simulink model "she_pwm_c_Bridge"  (R2023b)
settings: Solver=ode23t  StartTime=0.0  StopTime=0.1  MaxStep=1e-6  RelTol=1e-3
model workspace (MAT data in the model file):
  Mf = 48
  Vdc = 48
  ang_converted = 0
  compare_levels = [0 0]
  f = 50
  fs = 48
values from neighbouring files (symbols this model uses):
  angle_levels = zeros(1,angles_no)    [she_pwm.m]
libraries: spsIGBTDiodeLib x20, spsDCVoltageSourceLib x5, simulink x2, spsCurrentMeasurementLib x1, spsSeriesRLCBranchLib x1, spsTHDLib x1, spsVoltageMeasurementLib x1, sps_lib x1
settings Model: Creator=ixale  LastModifiedBy=ixale
settings DataIOCC: ReturnWorkspaceOutputs=off

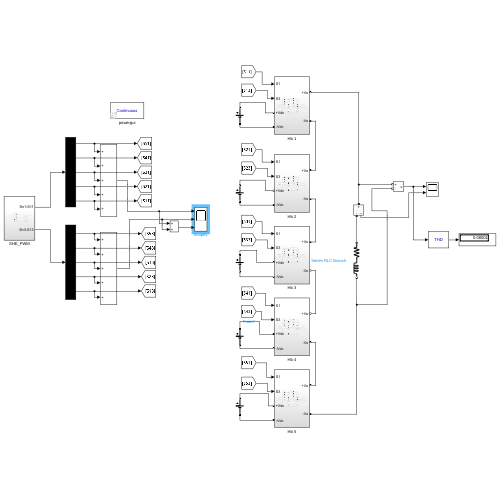
[thumbnail: Simulink's stored preview of the top-level diagram]
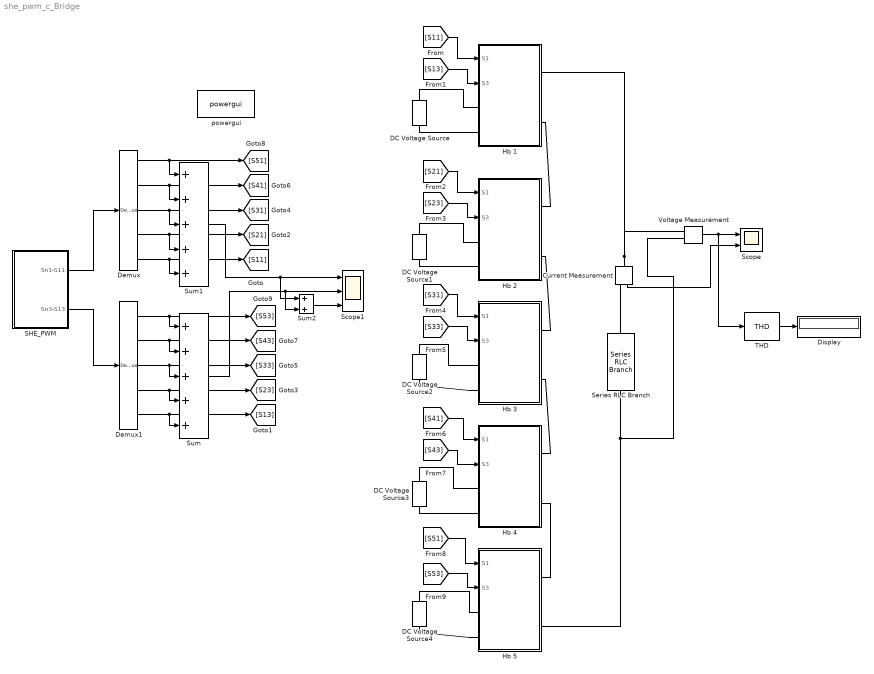
== system she_pwm_c_Bridge ==
  Current Measurement : spsCurrentMeasurementLib/Current Measurement  PhasorSimulation=off  OutputType=Complex  PSBequivalent=0
  DC Voltage Source{,1..4} (5 alike) : spsDCVoltageSourceLib/DC Voltage Source  Amplitude=Vdc  Measurements=None
  Demux : Demux  Outputs=5
  Demux1 : Demux  Outputs=5
  Display : Display
  Hb 1 : Subsystem
  Hb 2 : Subsystem
  Hb 3 : Subsystem
  Hb 4 : Subsystem
  Hb 5 : Subsystem
  SHE_PWM : Subsystem
  Scope : Scope  NumInputPorts=2
  Scope1 : Scope  NumInputPorts=3
  Series RLC Branch : spsSeriesRLCBranchLib/Series RLC Branch  LConnTagsString=__new0  RConnTagsString=__new0  BranchType=RL  Resistance=1  Inductance=1e-3  SetiL0=off  InitialCurrent=0  Capacitance=1e-6  Setx0=off  InitialVoltage=0  Measurements=None
  Sum : Sum  Inputs=+++++
  Sum1 : Sum  Inputs=+++++
  Sum2 : Sum
  THD : spsTHDLib/THD  Freq=50  Ts=0
  Voltage Measurement : spsVoltageMeasurementLib/Voltage Measurement  PhasorSimulation=off  OutputType=Complex  PSBequivalent=0
  powergui : sps_lib/powergui  Priority=1  SimulationMode=Continuous  SampleTime=1e-6  frequency=60  Iterations=50  frequencyindice=0  Pbase=100e6  ErrMax=1e-4  UnitsV=kV  UnitsW=MW  buscounter=0  FunctionMessages=off  echomessages=off  EnableUseOfTLC=off  CurrentSourceSwitches=off  DisableSnubberDevices=off  DisableRonSwitches=off  DisableVfSwitches=off  DisplayEquations=off  AutomaticDiscreteSolvers=off  SolverType=Tustin/Backward Euler (TBE)  Interpol=off  ExternalGateDelay=off  methode=off  Ts=100  x0status=blocks  SPID=on  SwTol=0  HookPort=off  NonlinearTolerance=1e-4  nMaxIteration=100  ContinueOnMaxIteration=off  RestoreLinks=warning  ResistiveCurrentMeasurement=off  Frange=[0:2:500]  Ylog=off  Xlog=on  ShowGrid=off  save=off  variable=ZData  structure=0  ZoomFFT=off  StartTime=0.0  cycles=1  DisplayStyle=1  fundamental=60  FreqAxis=off  MaxFrequency=1000  frequencyindicesteady=1  RmsSteady=1  display=off
  wires:
  Voltage Measurement/1 -> THD/1, Scope/1
  Current Measurement/1 -> Scope/2
  THD/1 -> Display/1
  [S11] -> Hb 1/1(S1)
  [S13] -> Hb 1/2(S3)
  [S23] -> Hb 2/2(S3)
  [S21] -> Hb 2/1(S1)
  [S31] -> Hb 3/1(S1)
  [S33] -> Hb 3/2(S3)
  [S43] -> Hb 4/2(S3)
  [S41] -> Hb 4/1(S1)
  [S51] -> Hb 5/1(S1)
  [S53] -> Hb 5/2(S3)
  SHE_PWM/1(Sn1-S11) -> Demux/1
  SHE_PWM/2(Sn3-S13) -> Demux1/1
  Demux1/3 -> Sum/3, [S33]
  Demux/1 -> Sum1/1, [S51]
  Demux/2 -> Sum1/2, [S41]
  Demux/3 -> Sum1/3, [S31]
  Demux/4 -> Sum1/4, [S21]
  Demux/5 -> Sum1/5, [S11]
  Sum1/1 -> Scope1/1, Sum2/1
  Sum/1 -> Sum2/2, Scope1/2
  Sum2/1 -> Scope1/3
  Demux1/4 -> Sum/4, [S23]
  Demux1/5 -> Sum/5, [S13]
  Demux1/2 -> Sum/2, [S43]
  Demux1/1 -> Sum/1, [S53]
  connections:
  Voltage Measurement/LConn2 -- Hb 5/RConn2 -- Series RLC Branch/RConn1
  Current Measurement/LConn1 -- Hb 1/RConn1 -- Voltage Measurement/LConn1
  Current Measurement/RConn1 -- Series RLC Branch/LConn1
  Hb 1/LConn1 -- DC Voltage Source/RConn1
  Hb 1/LConn2 -- DC Voltage Source/LConn1
  Hb 2/LConn1 -- DC Voltage Source1/RConn1
  Hb 2/LConn2 -- DC Voltage Source1/LConn1
  Hb 3/LConn1 -- DC Voltage Source2/RConn1
  Hb 3/LConn2 -- DC Voltage Source2/LConn1
  Hb 4/LConn1 -- DC Voltage Source3/RConn1
  Hb 4/LConn2 -- DC Voltage Source3/LConn1
  Hb 5/LConn1 -- DC Voltage Source4/RConn1
  Hb 5/LConn2 -- DC Voltage Source4/LConn1
  Hb 2/RConn1 -- Hb 1/RConn2
  Hb 3/RConn1 -- Hb 2/RConn2
  Hb 5/RConn1 -- Hb 4/RConn2
  Hb 4/RConn1 -- Hb 3/RConn2

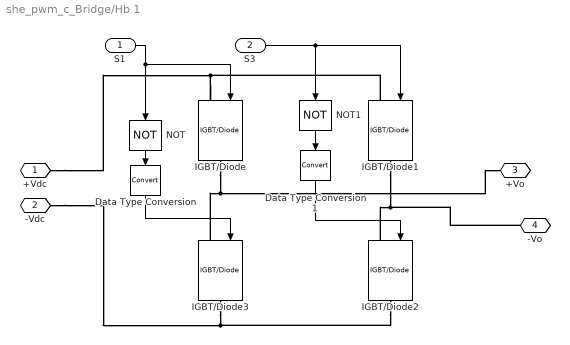
== system she_pwm_c_Bridge/Hb 1 ==
  S1 : Inport
  S3 : Inport  Port=2
  Data Type Conversion : DataTypeConversion  SaturateOnIntegerOverflow=off  RndMeth=Floor
  Data Type Conversion1 : DataTypeConversion  SaturateOnIntegerOverflow=off  RndMeth=Floor
  IGBT/Diode{,1..3} (4 alike) : spsIGBTDiodeLib/IGBT//Diode  Ron=1e-3  Rs=1e5  Cs=inf  Measurements=off
  NOT : Logic  Operator=NOT  IconShape=distinctive  AllPortsSameDT=off  OutDataTypeStr=boolean
  NOT1 : Logic  Operator=NOT  IconShape=distinctive  AllPortsSameDT=off  OutDataTypeStr=boolean
  +Vdc : PMIOPort  Side=Left
  -Vdc : PMIOPort  Port=2  Side=Left
  +Vo : PMIOPort  Port=3  Side=Right
  -Vo : PMIOPort  Port=4  Side=Right
  wires:
  S1/1 -> IGBT/Diode/1, NOT/1
  NOT/1 -> Data Type Conversion/1
  Data Type Conversion/1 -> IGBT/Diode3/1
  Data Type Conversion1/1 -> IGBT/Diode2/1
  NOT1/1 -> Data Type Conversion1/1
  S3/1 -> IGBT/Diode1/1, NOT1/1
  connections:
  IGBT/Diode3/RConn1 -- IGBT/Diode2/RConn1 -- -Vdc/RConn1
  IGBT/Diode1/LConn1 -- +Vdc/RConn1 -- IGBT/Diode/LConn1
  IGBT/Diode3/LConn1 -- IGBT/Diode/RConn1 -- +Vo/RConn1
  IGBT/Diode2/LConn1 -- IGBT/Diode1/RConn1 -- -Vo/RConn1

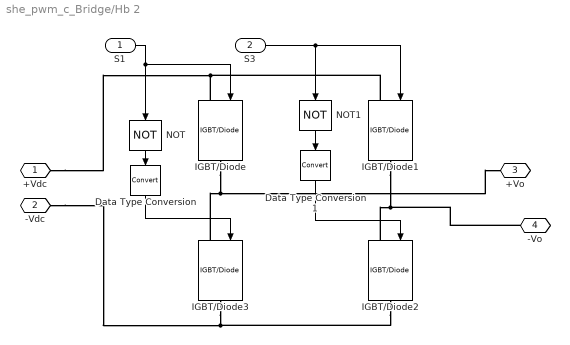
== system she_pwm_c_Bridge/Hb 2 ==
  S1 : Inport
  S3 : Inport  Port=2
  Data Type Conversion : DataTypeConversion  SaturateOnIntegerOverflow=off  RndMeth=Floor
  Data Type Conversion1 : DataTypeConversion  SaturateOnIntegerOverflow=off  RndMeth=Floor
  IGBT/Diode{,1..3} (4 alike) : spsIGBTDiodeLib/IGBT//Diode  Ron=1e-3  Rs=1e5  Cs=inf  Measurements=off
  NOT : Logic  Operator=NOT  IconShape=distinctive  AllPortsSameDT=off  OutDataTypeStr=boolean
  NOT1 : Logic  Operator=NOT  IconShape=distinctive  AllPortsSameDT=off  OutDataTypeStr=boolean
  +Vdc : PMIOPort  Side=Left
  -Vdc : PMIOPort  Port=2  Side=Left
  +Vo : PMIOPort  Port=3  Side=Right
  -Vo : PMIOPort  Port=4  Side=Right
  wires:
  S3/1 -> NOT1/1, IGBT/Diode1/1
  NOT1/1 -> Data Type Conversion1/1
  Data Type Conversion1/1 -> IGBT/Diode2/1
  Data Type Conversion/1 -> IGBT/Diode3/1
  NOT/1 -> Data Type Conversion/1
  S1/1 -> NOT/1, IGBT/Diode/1
  connections:
  IGBT/Diode1/RConn1 -- -Vo/RConn1 -- IGBT/Diode2/LConn1
  IGBT/Diode/RConn1 -- +Vo/RConn1 -- IGBT/Diode3/LConn1
  IGBT/Diode/LConn1 -- +Vdc/RConn1 -- IGBT/Diode1/LConn1
  IGBT/Diode2/RConn1 -- -Vdc/RConn1 -- IGBT/Diode3/RConn1

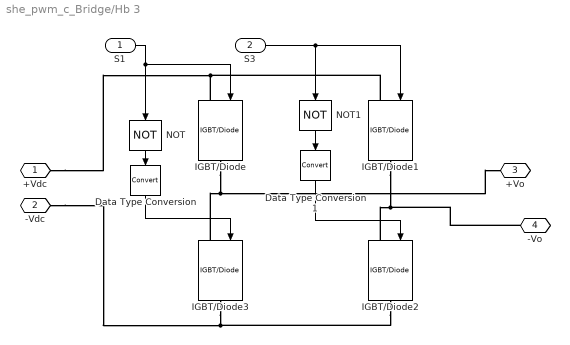
== system she_pwm_c_Bridge/Hb 3 ==
  S1 : Inport
  S3 : Inport  Port=2
  Data Type Conversion : DataTypeConversion  SaturateOnIntegerOverflow=off  RndMeth=Floor
  Data Type Conversion1 : DataTypeConversion  SaturateOnIntegerOverflow=off  RndMeth=Floor
  IGBT/Diode{,1..3} (4 alike) : spsIGBTDiodeLib/IGBT//Diode  Ron=1e-3  Rs=1e5  Cs=inf  Measurements=off
  NOT : Logic  Operator=NOT  IconShape=distinctive  AllPortsSameDT=off  OutDataTypeStr=boolean
  NOT1 : Logic  Operator=NOT  IconShape=distinctive  AllPortsSameDT=off  OutDataTypeStr=boolean
  +Vdc : PMIOPort  Side=Left
  -Vdc : PMIOPort  Port=2  Side=Left
  +Vo : PMIOPort  Port=3  Side=Right
  -Vo : PMIOPort  Port=4  Side=Right
  wires:
  S1/1 -> IGBT/Diode/1, NOT/1
  NOT/1 -> Data Type Conversion/1
  Data Type Conversion/1 -> IGBT/Diode3/1
  Data Type Conversion1/1 -> IGBT/Diode2/1
  NOT1/1 -> Data Type Conversion1/1
  S3/1 -> IGBT/Diode1/1, NOT1/1
  connections:
  IGBT/Diode3/RConn1 -- -Vdc/RConn1 -- IGBT/Diode2/RConn1
  IGBT/Diode1/LConn1 -- +Vdc/RConn1 -- IGBT/Diode/LConn1
  IGBT/Diode3/LConn1 -- +Vo/RConn1 -- IGBT/Diode/RConn1
  IGBT/Diode2/LConn1 -- -Vo/RConn1 -- IGBT/Diode1/RConn1

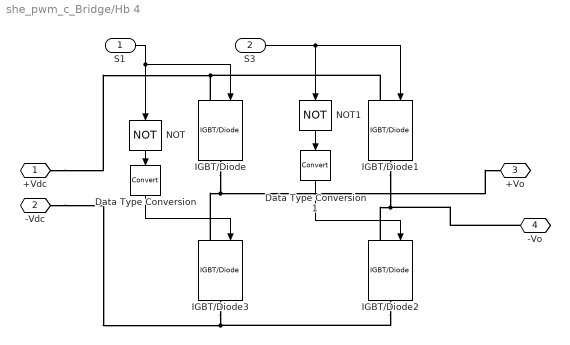
== system she_pwm_c_Bridge/Hb 4 ==
  S1 : Inport
  S3 : Inport  Port=2
  Data Type Conversion : DataTypeConversion  SaturateOnIntegerOverflow=off  RndMeth=Floor
  Data Type Conversion1 : DataTypeConversion  SaturateOnIntegerOverflow=off  RndMeth=Floor
  IGBT/Diode{,1..3} (4 alike) : spsIGBTDiodeLib/IGBT//Diode  Ron=1e-3  Rs=1e5  Cs=inf  Measurements=off
  NOT : Logic  Operator=NOT  IconShape=distinctive  AllPortsSameDT=off  OutDataTypeStr=boolean
  NOT1 : Logic  Operator=NOT  IconShape=distinctive  AllPortsSameDT=off  OutDataTypeStr=boolean
  +Vdc : PMIOPort  Side=Left
  -Vdc : PMIOPort  Port=2  Side=Left
  +Vo : PMIOPort  Port=3  Side=Right
  -Vo : PMIOPort  Port=4  Side=Right
  wires:
  S3/1 -> NOT1/1, IGBT/Diode1/1
  NOT1/1 -> Data Type Conversion1/1
  Data Type Conversion1/1 -> IGBT/Diode2/1
  Data Type Conversion/1 -> IGBT/Diode3/1
  NOT/1 -> Data Type Conversion/1
  S1/1 -> NOT/1, IGBT/Diode/1
  connections:
  IGBT/Diode1/RConn1 -- -Vo/RConn1 -- IGBT/Diode2/LConn1
  IGBT/Diode/RConn1 -- +Vo/RConn1 -- IGBT/Diode3/LConn1
  IGBT/Diode/LConn1 -- +Vdc/RConn1 -- IGBT/Diode1/LConn1
  IGBT/Diode2/RConn1 -- -Vdc/RConn1 -- IGBT/Diode3/RConn1

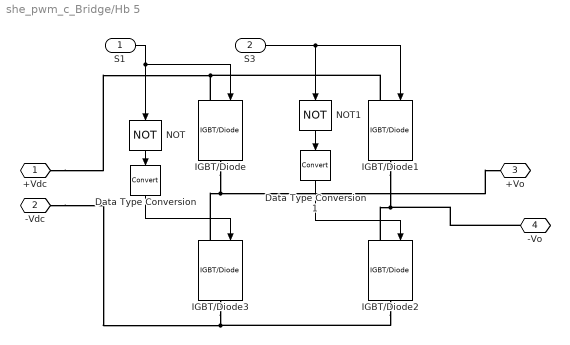
== system she_pwm_c_Bridge/Hb 5 ==
  S1 : Inport
  S3 : Inport  Port=2
  Data Type Conversion : DataTypeConversion  SaturateOnIntegerOverflow=off  RndMeth=Floor
  Data Type Conversion1 : DataTypeConversion  SaturateOnIntegerOverflow=off  RndMeth=Floor
  IGBT/Diode{,1..3} (4 alike) : spsIGBTDiodeLib/IGBT//Diode  Ron=1e-3  Rs=1e5  Cs=inf  Measurements=off
  NOT : Logic  Operator=NOT  IconShape=distinctive  AllPortsSameDT=off  OutDataTypeStr=boolean
  NOT1 : Logic  Operator=NOT  IconShape=distinctive  AllPortsSameDT=off  OutDataTypeStr=boolean
  +Vdc : PMIOPort  Side=Left
  -Vdc : PMIOPort  Port=2  Side=Left
  +Vo : PMIOPort  Port=3  Side=Right
  -Vo : PMIOPort  Port=4  Side=Right
  wires:
  S1/1 -> IGBT/Diode/1, NOT/1
  NOT/1 -> Data Type Conversion/1
  Data Type Conversion/1 -> IGBT/Diode3/1
  Data Type Conversion1/1 -> IGBT/Diode2/1
  NOT1/1 -> Data Type Conversion1/1
  S3/1 -> IGBT/Diode1/1, NOT1/1
  connections:
  IGBT/Diode3/RConn1 -- -Vdc/RConn1 -- IGBT/Diode2/RConn1
  IGBT/Diode1/LConn1 -- +Vdc/RConn1 -- IGBT/Diode/LConn1
  IGBT/Diode3/LConn1 -- +Vo/RConn1 -- IGBT/Diode/RConn1
  IGBT/Diode2/LConn1 -- -Vo/RConn1 -- IGBT/Diode1/RConn1

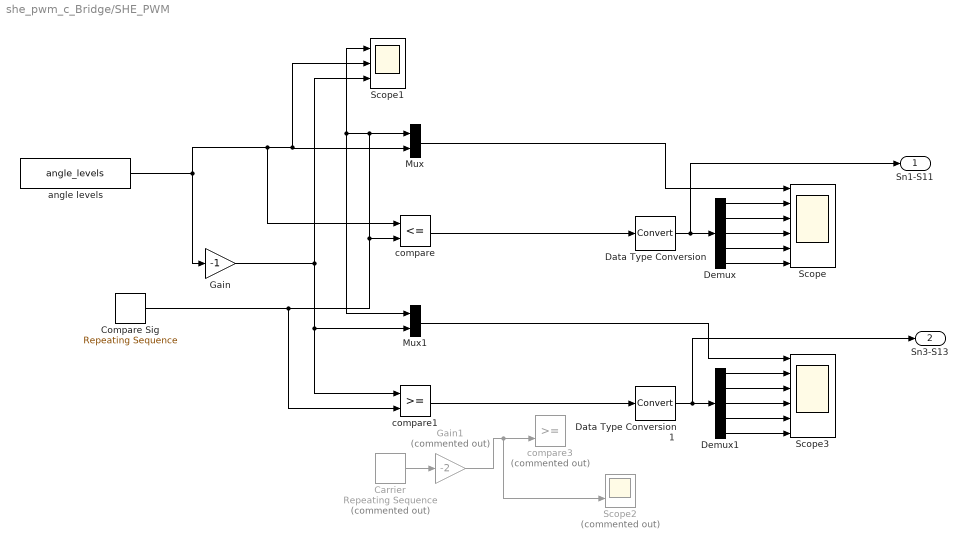
== system she_pwm_c_Bridge/SHE_PWM ==
  Carrier : simulink/Sources/Repeating Sequence  Commented=on  rep_seq_t=[0 0.5 1] * (1/(f*Mf))  rep_seq_y=[0 1 0]
  Compare Sig : simulink/Sources/Repeating Sequence  rep_seq_t=[0 0.25 0.5 0.75 1] * (1/(f))  rep_seq_y=[0 1 0 -1 0]
  Data Type Conversion : DataTypeConversion  SaturateOnIntegerOverflow=off  RndMeth=Floor
  Data Type Conversion1 : DataTypeConversion  SaturateOnIntegerOverflow=off  RndMeth=Floor
  Demux : Demux  Outputs=5
  Demux1 : Demux  Outputs=5
  Gain : Gain  Gain=-1
  Gain1 : Gain  Commented=on  Gain=-2
  Mux : Mux  Inputs=2
  Mux1 : Mux  Inputs=2
  Scope : Scope  NumInputPorts=6
  Scope1 : Scope  NumInputPorts=3
  Scope2 : Scope  Commented=on  NumInputPorts=2
  Scope3 : Scope  NumInputPorts=6
  angle levels : Constant  Value=angle_levels
  compare : RelationalOperator  Operator=<=  OutDataTypeStr=boolean  RndMeth=Simplest  InputSameDT=off
  compare1 : RelationalOperator  OutDataTypeStr=boolean  RndMeth=Simplest  InputSameDT=off
  compare3 : RelationalOperator  Commented=on  OutDataTypeStr=boolean  RndMeth=Simplest  InputSameDT=off
  Sn1-S11 : Outport
  Sn3-S13 : Outport  Port=2
  wires:
  Demux1/2 -> Scope3/3
  Demux1/5 -> Scope3/6
  Compare Sig/1 -> compare1/2, Mux1/1, Scope1/1, Mux/1, compare/2
  Mux/1 -> Scope/1
  angle levels/1 -> Scope1/2, Mux/2, compare/1, Gain/1
  Demux/4 -> Scope/5
  Demux/5 -> Scope/6
  Demux1/3 -> Scope3/4
  Demux1/4 -> Scope3/5
  Demux/3 -> Scope/4
  Demux/1 -> Scope/2
  Demux/2 -> Scope/3
  Gain/1 -> compare1/1, Mux1/2, Scope1/3
  Demux1/1 -> Scope3/2
  Mux1/1 -> Scope3/1
  Data Type Conversion/1 -> Sn1-S11/1, Demux/1
  Data Type Conversion1/1 -> Sn3-S13/1, Demux1/1
  Carrier/1 -> Gain1/1
  compare/1 -> Data Type Conversion/1
  Gain1/1 -> Scope2/2, compare3/2
  compare1/1 -> Data Type Conversion1/1
